simulink library "Lib_NM_JacobianCalc_TMATS"  (R2012b)
settings: Solver=ode45  StartTime=0.0  StopTime=10.0  RelTol=1e-3
Description:
  | Thomas Modules
settings Model: Creator=jwchapm2  LastModifiedBy=jwchapm2

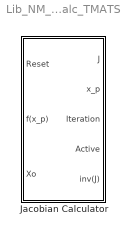
== system Lib_NM_JacobianCalc_TMATS ==
  Jacobian Calculator : Subsystem  mask(T-MATS: Jacobian Calculator Library Block){N_Per_M=[0.01; 0.05; 0.05]}
      mask prompts: N_Per_M "N_Per_M - Perturbations (mx1)"
      mask help: The Jacobian Calculator block calculates the Jabobian of the system by perturbing the system around an initial point and calculating the gradient for each perturbation. This module will run once on start up and then again only if the reset is pressed and can operatewith m inputs, where m is the number of independents in the system.
      mask Help: web(which('NumMthd_TMATS_JC.html'),'-helpbrowser')

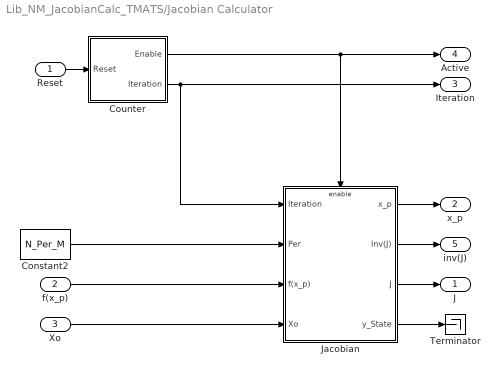
== system Lib_NM_JacobianCalc_TMATS/Jacobian Calculator ==
  Reset : Inport
  f(x_p) : Inport  Port=2
  Xo : Inport  Port=3
  Constant2 : Constant  Value=N_Per_M
  Counter : Subsystem  mask{N_Ind_M=length(N_Per_M)}
      mask prompts: N_Ind_M "number of independents, N_Ind_M"
  Jacobian : Subsystem
  Terminator : Terminator
  J : Outport
  x_p : Outport  Port=2
  Iteration : Outport  Port=3
  Active : Outport  Port=4
  inv(J) : Outport  Port=5
  wires:
  f(x_p)/1 -> Jacobian/3(f(x_p))
  Constant2/1 -> Jacobian/2(Per)
  Jacobian/1(x_p) -> x_p/1
  Reset/1 -> Counter/1(Reset)
  Counter/1(Enable) -> Active/1, Jacobian/Enable
  Xo/1 -> Jacobian/4(Xo)
  Counter/2(Iteration) -> Iteration/1, Jacobian/1(Iteration)
  Jacobian/2(Inv(J)) -> inv(J)/1
  Jacobian/3(J) -> J/1
  Jacobian/4(y_State) -> Terminator/1

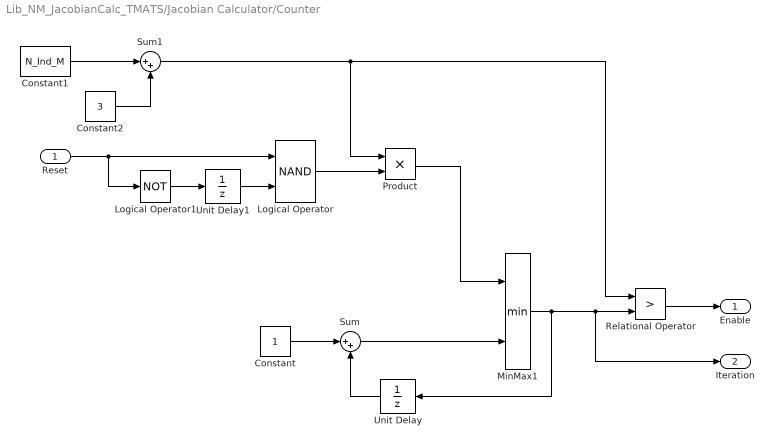
== system Lib_NM_JacobianCalc_TMATS/Jacobian Calculator/Counter ==
  Reset : Inport
  Constant : Constant
  Constant1 : Constant  Value=N_Ind_M
  Constant2 : Constant  Value=3
  Logical Operator : Logic  Operator=NAND  AllPortsSameDT=off  OutDataTypeStr=boolean
  Logical Operator1 : Logic  Operator=NOT  AllPortsSameDT=off  OutDataTypeStr=boolean
  MinMax1 : MinMax  Inputs=2
  Product : Product  RndMeth=Zero
  Relational Operator : RelationalOperator  Operator=>  OutDataTypeStr=boolean
  Sum : Sum  Inputs=|++
  Sum1 : Sum  Inputs=|++
  Unit Delay : UnitDelay  SampleTime=-1
  Unit Delay1 : UnitDelay  SampleTime=-1
  Enable : Outport
  Iteration : Outport  Port=2
  wires:
  Constant/1 -> Sum/1
  Product/1 -> MinMax1/1
  Sum/1 -> MinMax1/2
  Unit Delay/1 -> Sum/2
  MinMax1/1 -> Unit Delay/1, Iteration/1, Relational Operator/2
  Relational Operator/1 -> Enable/1
  Logical Operator/1 -> Product/2
  Reset/1 -> Logical Operator/1, Logical Operator1/1
  Logical Operator1/1 -> Unit Delay1/1
  Unit Delay1/1 -> Logical Operator/2
  Sum1/1 -> Relational Operator/1, Product/1
  Constant2/1 -> Sum1/2
  Constant1/1 -> Sum1/1

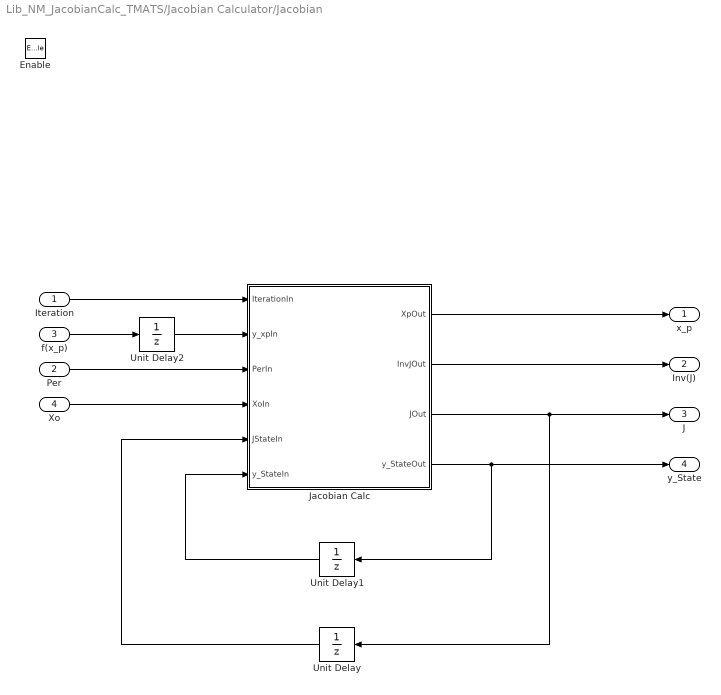
== system Lib_NM_JacobianCalc_TMATS/Jacobian Calculator/Jacobian ==
  Iteration : Inport
  Per : Inport  Port=2
  f(x_p) : Inport  Port=3
  Xo : Inport  Port=4
  Enable : EnablePort
  Jacobian Calc : MATLAB Function  TreatAsAtomicUnit=on
  Unit Delay : UnitDelay  InitialCondition=zeros(length(N_Per_M),length(N_Per_M))  SampleTime=-1
  Unit Delay1 : UnitDelay  InitialCondition=zeros(length(N_Per_M),length(N_Per_M)+1)  SampleTime=-1
  Unit Delay2 : UnitDelay  InitialCondition=zeros(length(N_Per_M),1)  SampleTime=-1
  x_p : Outport
  Inv(J) : Outport  Port=2
  J : Outport  Port=3
  y_State : Outport  Port=4
  wires:
  Jacobian Calc/1(XpOut) -> x_p/1
  Xo/1 -> Jacobian Calc/4(XoIn)
  Per/1 -> Jacobian Calc/3(PerIn)
  Iteration/1 -> Jacobian Calc/1(IterationIn)
  Jacobian Calc/3(JOut) -> Unit Delay/1, J/1
  Jacobian Calc/2(InvJOut) -> Inv(J)/1
  Unit Delay/1 -> Jacobian Calc/5(JStateIn)
  Jacobian Calc/4(y_StateOut) -> y_State/1, Unit Delay1/1
  Unit Delay1/1 -> Jacobian Calc/6(y_StateIn)
  f(x_p)/1 -> Unit Delay2/1
  Unit Delay2/1 -> Jacobian Calc/2(y_xpIn)

== matlab function Lib_NM_JacobianCalc_TMATS/Jacobian Calculator/Jacobian/Jacobian Calc ==
  data: IterationIn input; XpOut output; y_xpIn input; PerIn input; XoIn input; InvJOut output; JOut output; JStateIn input; y_StateIn input; y_StateOut output
function [XpOut, InvJOut, JOut, y_StateOut] = fcn(IterationIn, y_xpIn, PerIn, XoIn, JStateIn, y_StateIn)

% Set inital condiations
i = IterationIn;
XpOut = XoIn';
InvJOut = zeros(length(XoIn));
JOut = JStateIn;
y_StateOut = y_StateIn;
% Begin taking data from f(x) at iteration a+1
a = 1;
% Begin determining Jacobian at iteration b+1
b = a+1;

% Set Xp Output
if i > a && i <= length(XoIn) + a
    XpOut(i-a) = XpOut(i-a) + PerIn(i - a);
end

% setup state feedback
if length(XoIn) == 1
    if i == b;
        y_StateOut(1) = y_xpIn;
    end
else
    if i > a && i<= length(XoIn) + a+1;
        y_StateOut(:,i - a) = y_xpIn;
    end
end
% Create Jacobian
if i > b && i <= length(XoIn) + b
    if length(XoIn) == 1
        JOut = (y_xpIn - y_StateIn(1))/PerIn(1);
    else
        JOut(:,i - b) = (y_xpIn - y_StateOut(:,1))/PerIn(i - b);
    end
    if i == length(XoIn) + b
        if rank(JOut) == length(InvJOut)
            InvJOut = inv(JOut(:,:));
        else
            error('Jacobian can not be inverted.');
        end
    end
end
